simulink model "Logical_Operator"  (R2023b)
settings: Solver=VariableStepAuto  StartTime=0.0  StopTime=10.0  RelTol=1e-3
libraries: simulink x12
settings Model: Creator=hp  LastModifiedBy=hp

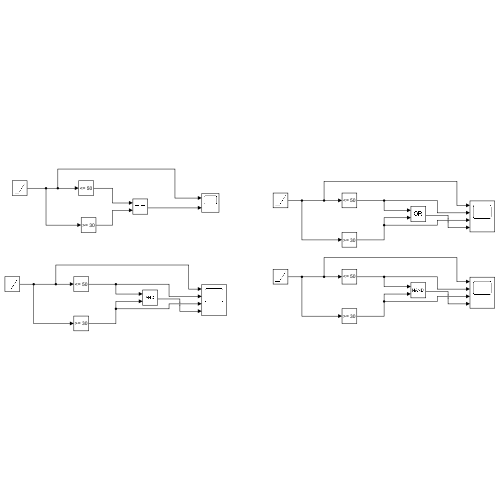
[thumbnail: Simulink's stored preview of the top-level diagram]
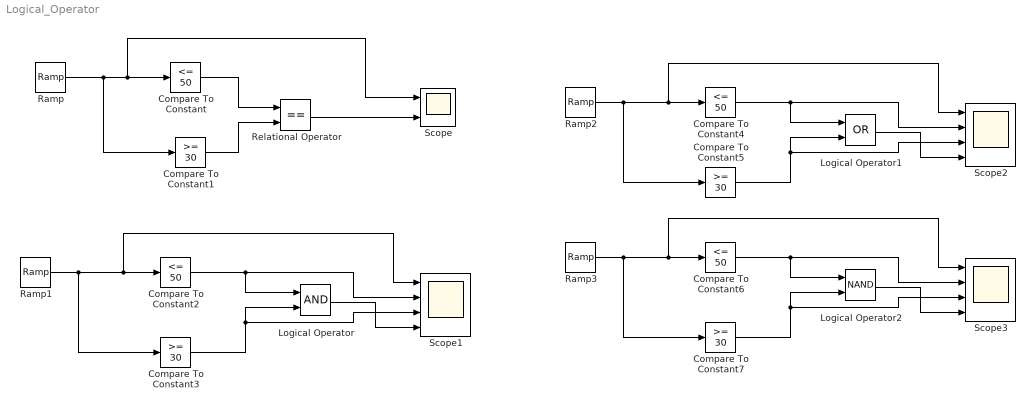
== system Logical_Operator ==
  Compare To Constant{,2,4,6} (4 alike) : simulink/Logic and Bit Operations/Compare To Constant  relop=<=  const=50  OutDataTypeStr=boolean
  Compare To Constant{1,3,5,7} (4 alike) : simulink/Logic and Bit Operations/Compare To Constant  relop=>=  const=30  OutDataTypeStr=boolean
  Logical Operator : Logic  AllPortsSameDT=off  OutDataTypeStr=boolean
  Logical Operator1 : Logic  Operator=OR  AllPortsSameDT=off  OutDataTypeStr=boolean
  Logical Operator2 : Logic  Operator=NAND  AllPortsSameDT=off  OutDataTypeStr=boolean
  Ramp{,1..3} (4 alike) : simulink/Sources/Ramp  slope=1  start=0  InitialOutput=27
  Relational Operator : RelationalOperator  Operator===  OutDataTypeStr=boolean  RndMeth=Simplest  InputSameDT=off
  Scope : Scope  NumInputPorts=2
  Scope1 : Scope  NumInputPorts=4
  Scope2 : Scope  NumInputPorts=4
  Scope3 : Scope  NumInputPorts=4
  wires:
  Ramp/1 -> Compare To Constant1/1, Scope/1, Compare To Constant/1
  Compare To Constant/1 -> Relational Operator/1
  Compare To Constant1/1 -> Relational Operator/2
  Relational Operator/1 -> Scope/2
  Ramp1/1 -> Compare To Constant3/1, Scope1/1, Compare To Constant2/1
  Compare To Constant2/1 -> Scope1/2, Logical Operator/1
  Compare To Constant3/1 -> Scope1/3, Logical Operator/2
  Logical Operator/1 -> Scope1/4
  Logical Operator1/1 -> Scope2/4
  Compare To Constant5/1 -> Logical Operator1/2, Scope2/3
  Compare To Constant4/1 -> Logical Operator1/1, Scope2/2
  Ramp2/1 -> Compare To Constant4/1, Scope2/1, Compare To Constant5/1
  Ramp3/1 -> Compare To Constant7/1, Scope3/1, Compare To Constant6/1
  Compare To Constant6/1 -> Scope3/2, Logical Operator2/1
  Compare To Constant7/1 -> Scope3/3, Logical Operator2/2
  Logical Operator2/1 -> Scope3/4
